simulink model "week2_3"  (R2020b)
settings: Solver=VariableStepAuto  StartTime=0.0  StopTime=10.0  RelTol=1e-3
settings Model: Creator=MY lenovo  LastModifiedBy=MY lenovo

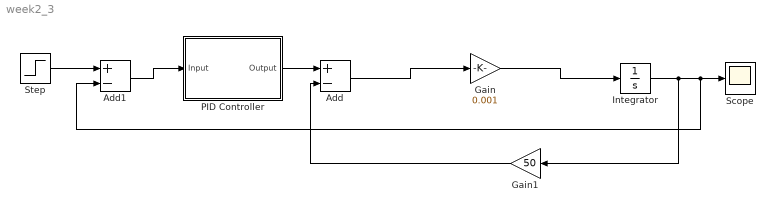
== system week2_3 ==
  Add : Sum  Inputs=+-
  Add1 : Sum  Inputs=+-
  Gain : Gain  Gain=0.001
  Gain1 : Gain  Gain=50
  Integrator : Integrator
  PID Controller : Subsystem
  Scope : Scope
  Step : Step  SampleTime=0
  wires:
  Gain/1 -> Integrator/1
  Gain1/1 -> Add/2
  PID Controller/1(Output) -> Add/1
  Add/1 -> Gain/1
  Step/1 -> Add1/1
  Add1/1 -> PID Controller/1(Input)
  Integrator/1 -> Add1/2, Scope/1, Gain1/1

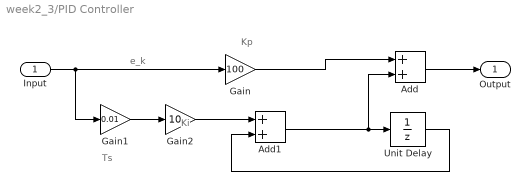
== system week2_3/PID Controller ==
  note: Ki
  note: Kp
  note: Ts
  note: e_k
  Input : Inport
  Add : Sum
  Add1 : Sum
  Gain : Gain  Gain=100
  Gain1 : Gain  Gain=0.01
  Gain2 : Gain  Gain=10
  Unit Delay : UnitDelay  SampleTime=-1  HasFrameUpgradeWarning=on
  Output : Outport
  wires:
  Input/1 -> Gain1/1, Gain/1
  Gain/1 -> Add/1
  Add/1 -> Output/1
  Gain1/1 -> Gain2/1
  Gain2/1 -> Add1/1
  Add1/1 -> Add/2, Unit Delay/1
  Unit Delay/1 -> Add1/2
